simulink model "vehicle_model_traction"  (R2018a)
settings: Solver=VariableStepAuto  StartTime=0.0  StopTime=10.0  RelTol=1e-3
libraries: simulink x1, qss_tb_library x1
settings Model: Creator=Luís Miranda  LastModifiedBy=Luís Miranda

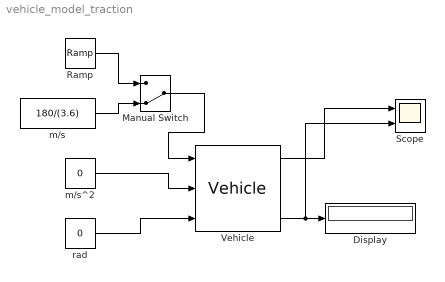
== system vehicle_model_traction ==
  Display : Display
  Manual Switch : ManualSwitch  CurrentSetting=0
  Ramp : simulink/Sources/Ramp  slope=5/3.6/10  start=0  InitialOutput=0
  Scope : Scope  NumInputPorts=2
  Vehicle : qss_tb_library/Vehicle/Vehicle  Tag=vehicle  m_f=1250  A_f=2.1  cw=0.31  mu=0.01  k_inertia=5
  m/s : Constant  Value=180/(3.6)
  m/s^2 : Constant  Value=0
  rad : Constant  Value=0
  wires:
  rad/1 -> Vehicle/3
  m/s^2/1 -> Vehicle/2
  m/s/1 -> Manual Switch/2
  Vehicle/3 -> Scope/2, Display/1
  Vehicle/1 -> Scope/1
  Ramp/1 -> Manual Switch/1
  Manual Switch/1 -> Vehicle/1
